simulink model "drive_model2_2021"  (R2022a)
settings: Solver=VariableStepAuto  StartTime=0.0  StopTime=10.0  RelTol=1e-3
libraries: spsMosfetLib x6, spsSeriesRLCBranchLib x3, spsPermanentMagnetSynchronousMachineLib x1, spsThreePhaseSourceLib x1, spsUniversalBridgeLib x1, spspowerguiLib x1
settings Model: Creator=Goktug  LastModifiedBy=Goktug

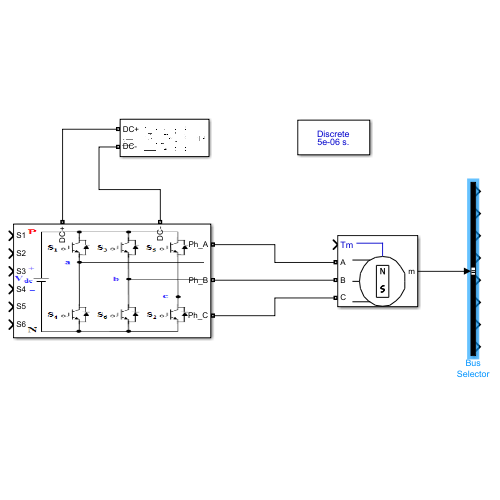
[thumbnail: Simulink's stored preview of the top-level diagram]
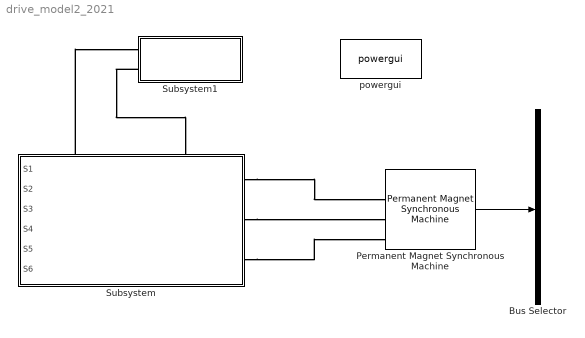
== system drive_model2_2021 ==
  Bus Selector : BusSelector  OutputSignals=Rotor speed wm (rad/s),Stator current is_a (A),Stator current is_b (A),Stator current is_c (A),Stator current is_q (A),Stator current is_d (A),Electromagnetic torque Te (N*m),Rotor angle thetam (rad)
  Permanent Magnet Synchronous Machine : spsPermanentMagnetSynchronousMachineLib/Permanent Magnet Synchronous Machine  NbPhases=3  FluxDistribution=Sinusoidal  RotorType=Round  MechanicalLoad=Torque Tm  PresetModel=No  ShowDetailedParameters=on  MeasurementBus=off  Resistance=16e-3  Inductance=8.5e-3  dqInductances=[8.5e-3,8.5e-3]  La=165e-6  MachineConstant=Flux linkage established by magnets (V.s)  Flux=0.11  VoltageCst=159.6143  TorqueCst=1.32  Flat=120  Mechanical=[0.5 0 8 0]  PolePairs=4  InitialConditions=[0,0, 0,0]  InitialConditions5ph=[0 0 0 0 0 0]  RefAngle=90 degrees behind phase A axis (modified Park)  IterativeDiscreteModel=Trapezoidal non iterative  TsBlock=-1  TsPowergui=0
  Subsystem : Subsystem
      settings: PortSchema="{\"entries\":[{\"content\":{\"sides\":[{\"content\":{\"connectorIds\":[\"In1\",\"In2\",\"In3\",\"In4\",\"In5\",\"In6\"]},\"type\":\"ConnectorPlacement.EquallySpacedRectSide\",\"uuid\":\"7f4ea820-4c70-4af6-9af4-0b0f241e3ef1\"},{\"content\":{\"connectorIds\":[\"RConn1\",\"RConn2\",\"RConn3\"],\"side\":\"RIGHT\"},\"type\":\"ConnectorPlacement.EquallySpacedRectSide\",\"uuid\":\"773c8554-3ddc-44eb-9c7e-8e31c6a64932\"},{\"content\":{\"connectorIds\":[\"LConn1\",\"LConn2\"],\"side\":\"TOP\"},\"type\":\"ConnectorPlacement.EquallySpacedRectSide\",\"uuid\":\"b69331c1-3701-4f00-ae63-6be74d84d27f\"}]},\"type\":\"ConnectorPlacement.EquallySpacedConnector\",\"uuid\":\"8208b667-ecd4-4b99-b733-c445d2b47d27\"}],\"packageUris\":[\"http://schema.mathworks.com/mf0/Connector/R2020b\"],\"version\":\"1.0\"}"
      mask Display: image('$imagefile'); % Use "Edit Image" on toolstrip to change.
  Subsystem1 : Subsystem
      mask Display: image('filter.PNG'); % Use "Edit Image" on toolstrip to change.
  powergui : spspowerguiLib/powergui  Priority=1  SimulationMode=Discrete  SampleTime=5e-6  frequency=60  Iterations=50  frequencyindice=0  Pbase=100e6  ErrMax=1e-4  UnitsV=kV  UnitsW=MW  buscounter=0  FunctionMessages=off  echomessages=off  EnableUseOfTLC=off  CurrentSourceSwitches=off  DisableSnubberDevices=off  DisableRonSwitches=off  DisableVfSwitches=off  DisplayEquations=off  AutomaticDiscreteSolvers=off  SolverType=Tustin/Backward Euler (TBE)  Interpol=off  ExternalGateDelay=off  methode=off  Ts=100  x0status=blocks  SPID=on  SwTol=0  HookPort=off  NonlinearTolerance=1e-4  nMaxIteration=100  ContinueOnMaxIteration=off  RestoreLinks=warning  ResistiveCurrentMeasurement=off  Frange=[0:2:500]  Ylog=off  Xlog=on  ShowGrid=off  save=off  variable=ZData  structure=0  ZoomFFT=off  StartTime=0.0  cycles=1  DisplayStyle=1  fundamental=60  FreqAxis=off  MaxFrequency=1000  frequencyindicesteady=1  RmsSteady=1  display=off
  wires:
  Permanent Magnet Synchronous Machine/1 -> Bus Selector/1
  connections:
  Subsystem1/RConn2 -- Subsystem/LConn2
  Subsystem/LConn1 -- Subsystem1/RConn1
  Subsystem/RConn1 -- Permanent Magnet Synchronous Machine/LConn1
  Subsystem/RConn2 -- Permanent Magnet Synchronous Machine/LConn2
  Subsystem/RConn3 -- Permanent Magnet Synchronous Machine/LConn3

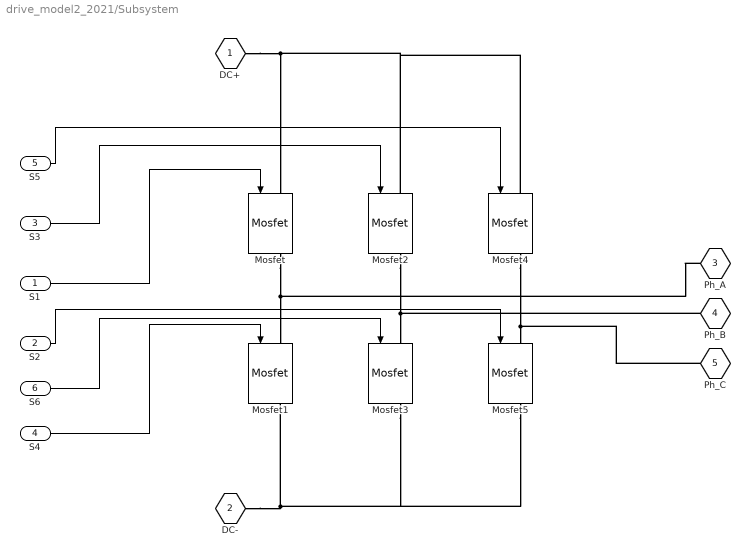
== system drive_model2_2021/Subsystem ==
  S1 : Inport
  S2 : Inport  Port=2
  S3 : Inport  Port=3
  S4 : Inport  Port=4
  S5 : Inport  Port=5
  S6 : Inport  Port=6
  Mosfet{,1..5} (6 alike) : spsMosfetLib/Mosfet  Ron=0.1  Lon=0  Rd=0.01  Vfd=0  IC=0  Rs=1e5  Cs=inf  Measurements=on
  DC+ : PMIOPort  Side=Left
  DC- : PMIOPort  Port=2  Side=Left
  Ph_A : PMIOPort  Port=3  Side=Right
  Ph_B : PMIOPort  Port=4  Side=Right
  Ph_C : PMIOPort  Port=5  Side=Right
  wires:
  S1/1 -> Mosfet/1
  S3/1 -> Mosfet2/1
  S5/1 -> Mosfet4/1
  S4/1 -> Mosfet1/1
  S6/1 -> Mosfet3/1
  S2/1 -> Mosfet5/1
  connections:
  Mosfet/RConn1 -- Ph_A/RConn1 -- Mosfet1/LConn1
  Mosfet2/RConn1 -- Ph_B/RConn1 -- Mosfet3/LConn1
  Mosfet4/RConn1 -- Ph_C/RConn1 -- Mosfet5/LConn1
  DC-/RConn1 -- Mosfet5/RConn1 -- Mosfet3/RConn1 -- Mosfet1/RConn1
  DC+/RConn1 -- Mosfet4/LConn1 -- Mosfet2/LConn1 -- Mosfet/LConn1

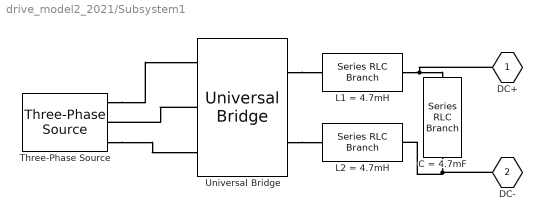
== system drive_model2_2021/Subsystem1 ==
  C = 4.7mF : spsSeriesRLCBranchLib/Series RLC Branch  LConnTagsString=__new0  RConnTagsString=__new0  BranchType=RC  Resistance=1e-6  Inductance=1e-3  SetiL0=off  InitialCurrent=0  Capacitance=4.7e-3  Setx0=off  InitialVoltage=0  Measurements=None
  L1 = 4.7mH : spsSeriesRLCBranchLib/Series RLC Branch  LConnTagsString=__new0  RConnTagsString=__new0  BranchType=RL  Resistance=1e-6  Inductance=4.7e-3  SetiL0=off  InitialCurrent=0  Capacitance=1e-6  Setx0=off  InitialVoltage=0  Measurements=None
  L2 = 4.7mH : spsSeriesRLCBranchLib/Series RLC Branch  LConnTagsString=__new0  RConnTagsString=__new0  BranchType=RL  Resistance=1e-6  Inductance=4.7e-3  SetiL0=off  InitialCurrent=0  Capacitance=1e-6  Setx0=off  InitialVoltage=0  Measurements=None
  Three-Phase Source : spsThreePhaseSourceLib/Three-Phase Source  InternalConnection=Yg  VoltagePhases=off  Voltage=400  PhaseAngle=0  Voltage_phases=[25e3 25e3 25e3]/sqrt(3)  PhaseAngles_phases=[0 -120 +120]  Frequency=50  NonIdealSource=off  SpecifyImpedance=off  Resistance=0.8929  Inductance=16.58e-3  ShortCircuitLevel=100e6  BaseVoltage=25e3  XRratio=7  BusType=swing  Pref=10e3  Qref=0  Prefabc=[10e3, 10e3, 10e3]  Qrefabc=[0, 0, 0]  Qmin=-inf  Qmax=inf
  Universal Bridge : spsUniversalBridgeLib/Universal Bridge  Arms=3  SnubberResistance=1e5  SnubberCapacitance=inf  Device=Diodes  Ron=1e-3  Lon=0  ForwardVoltages="[  0  0  ]"  ForwardVoltage=0  GTOparameters=[ 10e-6 , 20e-6 ]  IGBTparameters=[ 1e-6 , 2e-6 ]  Measurements=None  Measurements_2=None  converterType=Rectifier
  DC+ : PMIOPort  Side=Right
  DC- : PMIOPort  Port=2  Side=Right
  connections:
  Universal Bridge/RConn1 -- L1 = 4.7mH/LConn1
  Three-Phase Source/RConn3 -- Universal Bridge/LConn3
  C = 4.7mF/RConn1 -- DC-/RConn1 -- L2 = 4.7mH/RConn1
  Universal Bridge/RConn2 -- L2 = 4.7mH/LConn1
  Three-Phase Source/RConn1 -- Universal Bridge/LConn1
  Universal Bridge/LConn2 -- Three-Phase Source/RConn2
  L1 = 4.7mH/RConn1 -- DC+/RConn1 -- C = 4.7mF/LConn1
